simulink model "CODE_GEN"  (R2023b)
settings: Solver=FixedStepDiscrete  StartTime=0.0  StopTime=10.0  FixedStep=0.001  RelTol=1e-3
values from neighbouring files (symbols this model uses):
  alpha = 15/180*pi    (= 0.261799387799)    [MPC_HAC_simulation.m]    (also in init_HAC_simulation.m)
  beta = 50/180*pi    (= 0.872664625997)    [MPC_HAC_simulation.m]    (also in init_HAC_simulation.m)
  E_up = m*g*L*cos(0)    [init_HAC_simulation.m]    (also in init_model.m)
  eta = 1.3    [init_HAC_simulation.m]    (also in init_model.m)
  g = [g; st_next - st_next_RK4]    [MPC_cartPend_casadi.m]    (also in MPC_cartPend_casadi_scaled.m; MPC_casadi_block.m; continuous_cartpend.m = 9.80665; init_HAC_simulation.m = 9.80665)
  I = 8.7395e-04    (= 0.00087395)    [MPC_casadi_block.m]    (also in continuous_cartpend.m = 0.0008739525; init_HAC_simulation.m = 0.0008739525; init_MPC.m = 0.0008739525; init_NMPC.m = 0.0008739525)
  k_cw = 6    [init_HAC_simulation.m]    (also in init_model.m)
  k_em = 10    [init_HAC_simulation.m]    (also in init_model.m)
  k_su = 2    [init_HAC_simulation.m]    (also in init_model.m)
  k_vw = 2.5    [init_HAC_simulation.m]    (also in init_model.m)
  L = 0.1500    (= 0.15)    [MPC_casadi_block.m]    (also in continuous_cartpend.m; init_HAC_simulation.m; init_MPC.m; init_NMPC.m)
  m = 0.116527    [MPC_casadi_block.m]    (also in continuous_cartpend.m; init_HAC_simulation.m; init_MPC.m; init_NMPC.m)
  q_max = 15/180*pi    (= 0.261799387799)    [MPC_HAC_simulation.m]    (also in MPC_cartPend_casadi.m = inf; MPC_cartPend_casadi_scaled.m = 6.28318530718; MPC_casadi_block.m = inf; init_HAC_simulation.m)
  q_min = -q_max    (= -0.261799387799)    [MPC_HAC_simulation.m]    (also in MPC_cartPend_casadi.m = -inf; MPC_cartPend_casadi_scaled.m = -6.28318530718; MPC_casadi_block.m = -inf; init_HAC_simulation.m)
  q_sqm = zeros(1, n_rules_q)    [MPC_HAC_simulation.m]    (also in init_HAC_simulation.m)
  qd_max = inf    [MPC_HAC_simulation.m]    (also in MPC_cartPend_casadi.m; MPC_cartPend_casadi_scaled.m = 13; MPC_casadi_block.m; init_HAC_simulation.m = 5)
  qd_min = -qd_max    (= -inf)    [MPC_HAC_simulation.m]    (also in MPC_cartPend_casadi.m; MPC_cartPend_casadi_scaled.m = -13; MPC_casadi_block.m; init_HAC_simulation.m = -5)
  qd_sqm = zeros(1, n_rules_qd)    [MPC_HAC_simulation.m]    (also in init_HAC_simulation.m)
  u_max = 3 * 9.80665    (= 29.41995)    [MPC_HAC_simulation.m]    (also in MPC_cartPend_casadi.m = 29.43; MPC_cartPend_casadi_scaled.m = 29.43; MPC_casadi_block.m = 29.43; init_HAC_simulation.m)
  u_min = -u_max    (= -29.41995)    [MPC_HAC_simulation.m]    (also in MPC_cartPend_casadi.m = -29.43; MPC_cartPend_casadi_scaled.m = -29.43; MPC_casadi_block.m = -29.43; init_HAC_simulation.m)
  u_q_sqm = zeros(1, n_rules_q)    [MPC_HAC_simulation.m]    (also in init_HAC_simulation.m)
  u_qd_sqm = zeros(1, n_rules_qd)    [MPC_HAC_simulation.m]    (also in init_HAC_simulation.m)
  u_x_sqm = zeros(1, n_rules_x)    [MPC_HAC_simulation.m]    (also in init_HAC_simulation.m)
  u_xd_sqm = zeros(1, n_rules_xd)    [MPC_HAC_simulation.m]    (also in init_HAC_simulation.m)
  uMax = 3*g    (= 29.41995)    [init_HAC_simulation.m]    (also in init_MPC.m; init_NMPC.m; init_model.m)
  w_high = 1    [MPC_HAC_simulation.m]    (also in init_HAC_simulation.m)
  w_low = 0.25    [MPC_HAC_simulation.m]    (also in init_HAC_simulation.m)
  x1_max = 0.43    [init_HAC_simulation.m]    (also in init_MPC.m; init_NMPC.m; init_model.m)
  x2_max = 2    [init_HAC_simulation.m]    (also in init_MPC.m; init_NMPC.m; init_model.m)
  x_max = 0.43    [MPC_HAC_simulation.m]    (also in MPC_cartPend_casadi.m; MPC_cartPend_casadi_scaled.m; MPC_casadi_block.m; init_HAC_simulation.m)
  x_min = -x_max    (= -0.43)    [MPC_HAC_simulation.m]    (also in MPC_cartPend_casadi.m; MPC_cartPend_casadi_scaled.m; MPC_casadi_block.m; init_HAC_simulation.m)
  x_sqm = zeros(1, n_rules_x)    [MPC_HAC_simulation.m]    (also in init_HAC_simulation.m; my_HAC.m = [0 0.00390625 0.0078125 0.01171875 0.015625 0.0234375 0.0312)
  xd_max = 2.0    (= 2)    [MPC_HAC_simulation.m]    (also in MPC_cartPend_casadi.m; MPC_cartPend_casadi_scaled.m; MPC_casadi_block.m; init_HAC_simulation.m)
  xd_min = -xd_max    (= -2)    [MPC_HAC_simulation.m]    (also in MPC_cartPend_casadi.m; MPC_cartPend_casadi_scaled.m; MPC_casadi_block.m; init_HAC_simulation.m)
  xd_sqm = zeros(1, n_rules_xd)    [MPC_HAC_simulation.m]    (also in init_HAC_simulation.m)
libraries: fuzblock x2
settings Model: Creator=doann  LastModifiedBy=doann
settings OptimizationCC: DefaultParameterBehavior=Inlined  UseDivisionForNetSlopeComputation=on  GainParamInheritBuiltInType=on  UseFloatMulNetSlope=on  InlineInvariantSignals=on  PassReuseOutputArgsAs=Individual arguments  ZeroExternalMemoryAtStartup=off  ZeroInternalMemoryAtStartup=off  NoFixptDivByZeroProtection=on  EfficientFloat2IntCast=on  LifeSpan=1  OptimizeBlockOrder=speed  DifferentSizesBufferReuse=on  EfficientTunableParamExpr=on
settings DebuggingCC: ParameterTunabilityLossMsg=error
settings HardwareCC: ProdBitPerPointer=32  ProdBitPerSizeT=32  ProdBitPerPtrDiffT=32  ProdLargestAtomicInteger=Long  ProdLargestAtomicFloat=Double  ProdWordSize=32  ProdLongLongMode=on  ProdHWDeviceType=ARM Compatible->ARM Cortex-M
settings SFSimCC: MATLABDynamicMemAlloc=off
settings RTWCC: Description=Embedded Coder  SystemTargetFile=ert.tlc  TemplateMakefile=ert_default_tmf  TargetLang=C++
settings CodeAppCC: ForceParamTrailComments=on  IgnoreCustomStorageClasses=off  OperatorAnnotations=on  SimulinkDataObjDesc=on  SFDataObjDesc=on  CustomSymbolStrGlobalVar=rt$N$M  CustomSymbolStrType=$N$M  CustomSymbolStrFcn=$N$M$F  CustomSymbolStrMacro=$N$M  InsertBlockDesc=on
settings ERTTargetCC: TargetLangStandard=C++11 (ISO)  GenerateSampleERTMain=on  IncludeMdlTerminateFcn=off  CombineSignalStateStructs=on  SupportAbsoluteTime=off  CodeInterfacePackaging=C++ class  SupportComplex=off  SupportNonInlinedSFcns=on  InlinedParameterPlacement=NonHierarchical  RootIOFormat=Structure reference  ERTCustomFileTemplate=example_file_process.tlc  ERTFilePackagingFormat=CompactWithDataFile

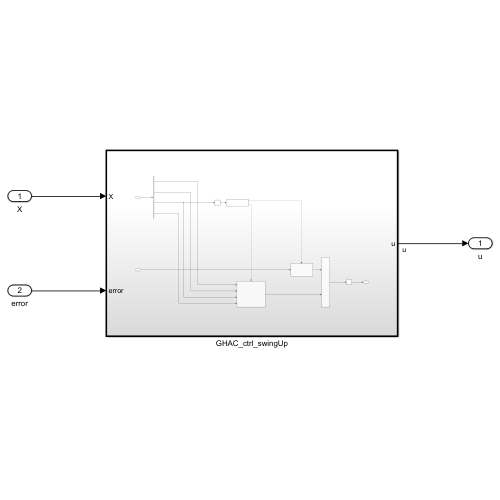
[thumbnail: Simulink's stored preview of the top-level diagram]
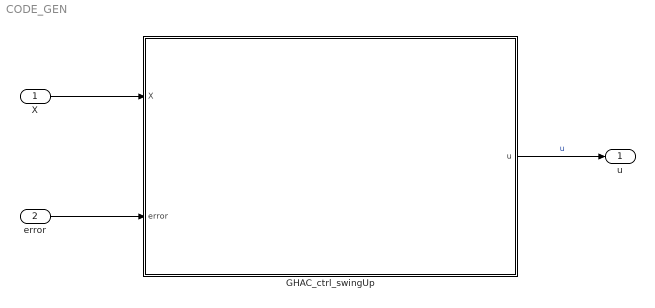
== system CODE_GEN ==
  X : Inport
  error : Inport  Port=2
  GHAC_ctrl_swingUp : Subsystem  TreatAsAtomicUnit=on  SystemSampleTime=0.001
  u : Outport
  wires:
  GHAC_ctrl_swingUp/1(u) -> u/1  "u"
  X/1 -> GHAC_ctrl_swingUp/1(X)
  error/1 -> GHAC_ctrl_swingUp/2(error)

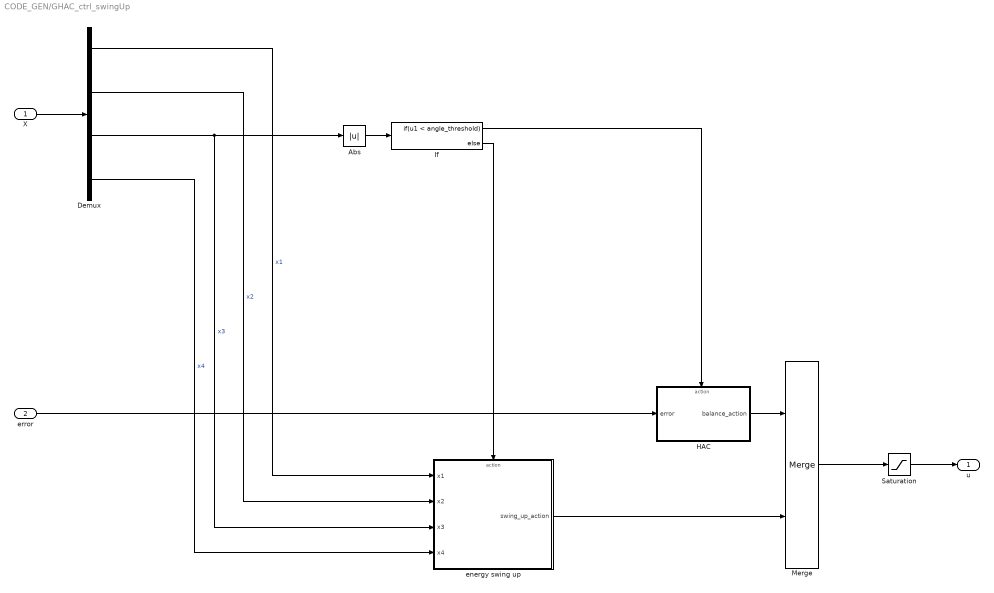
== system CODE_GEN/GHAC_ctrl_swingUp ==
  X : Inport
  error : Inport  Port=2
  Abs : Abs  SaturateOnIntegerOverflow=off
  Demux : Demux
  HAC : Subsystem  TreatAsAtomicUnit=on
  If : If  IfExpression=u1 < angle_threshold
  Merge : Merge
  Saturation : Saturate  UpperLimit=uMax  LowerLimit=-uMax
  energy swing up : Subsystem  TreatAsAtomicUnit=on
  u : Outport
  wires:
  X/1 -> Demux/1
  Demux/3 -> Abs/1, energy swing up/3(x3)  "x3"
  Demux/4 -> energy swing up/4(x4)  "x4"
  Abs/1 -> If/1
  If/1 -> HAC/Action
  If/2 -> energy swing up/Action
  HAC/1(balance_action) -> Merge/1
  energy swing up/1(swing_up_action) -> Merge/2
  error/1 -> HAC/1(error)
  Demux/2 -> energy swing up/2(x2)  "x2"
  Demux/1 -> energy swing up/1(x1)  "x1"
  Merge/1 -> Saturation/1
  Saturation/1 -> u/1

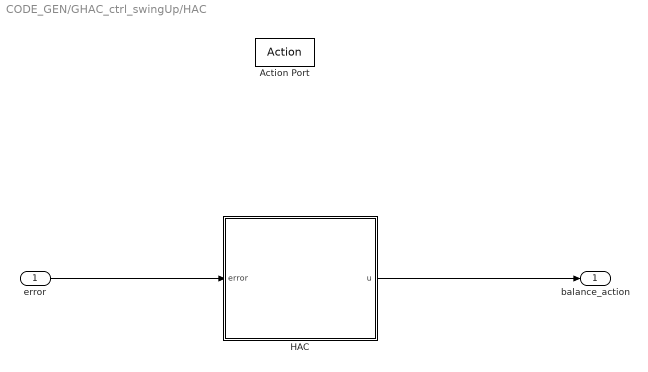
== system CODE_GEN/GHAC_ctrl_swingUp/HAC ==
  error : Inport
  Action Port : ActionPort  ActionPortLabel=if(u1 < angle_threshold)
  HAC : Subsystem
  balance_action : Outport
  wires:
  error/1 -> HAC/1(error)
  HAC/1(u) -> balance_action/1

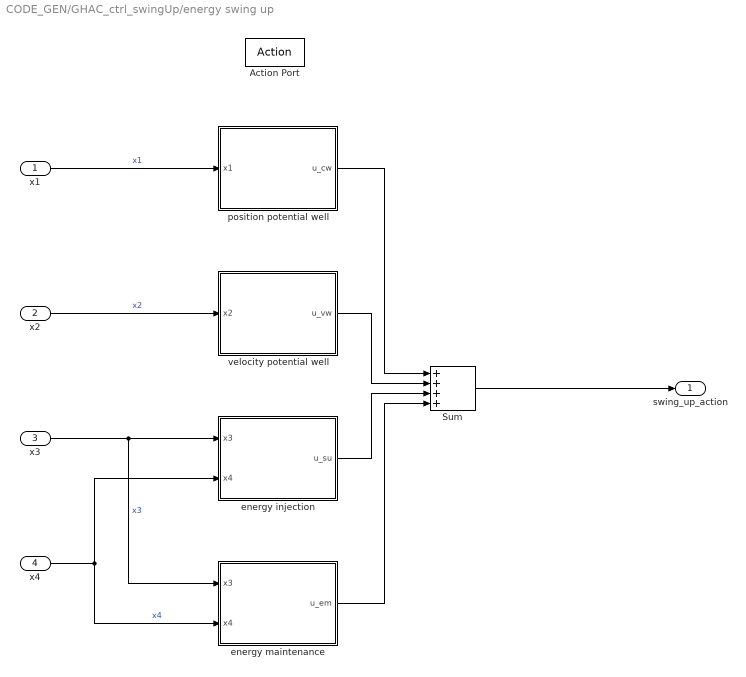
== system CODE_GEN/GHAC_ctrl_swingUp/energy swing up ==
  x1 : Inport
  x2 : Inport  Port=2
  x3 : Inport  Port=3
  x4 : Inport  Port=4
  Action Port : ActionPort  ActionPortLabel=else
  Sum : Sum  Inputs=++++
  energy injection : Subsystem
  energy maintenance : Subsystem
  position potential well : Subsystem
  velocity potential well : Subsystem
  swing_up_action : Outport
  wires:
  energy injection/1(u_su) -> Sum/3
  x2/1 -> velocity potential well/1(x2)  "x2"
  velocity potential well/1(u_vw) -> Sum/2
  Sum/1 -> swing_up_action/1
  energy maintenance/1(u_em) -> Sum/4
  x3/1 -> energy maintenance/1(x3), energy injection/1(x3)  "x3"
  x1/1 -> position potential well/1(x1)  "x1"
  x4/1 -> energy injection/2(x4), energy maintenance/2(x4)  "x4"
  position potential well/1(u_cw) -> Sum/1

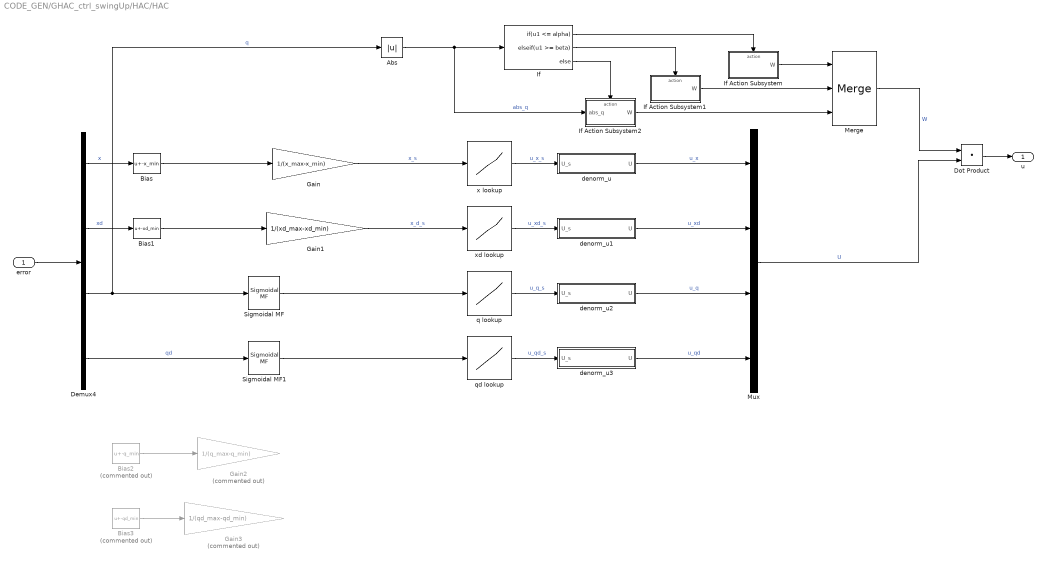
== system CODE_GEN/GHAC_ctrl_swingUp/HAC/HAC ==
  error : Inport
  Abs : Abs  SaturateOnIntegerOverflow=off
  Bias : Bias  Bias=-x_min  SaturateOnIntegerOverflow=off
  Bias1 : Bias  Bias=-xd_min  SaturateOnIntegerOverflow=off
  Bias2 : Bias  Commented=on  Bias=-q_min  SaturateOnIntegerOverflow=off
  Bias3 : Bias  Commented=on  Bias=-qd_min  SaturateOnIntegerOverflow=off
  Demux4 : Demux
  Dot Product : DotProduct  OutDataTypeStr=Inherit: Inherit via internal rule
  Gain : Gain  Gain=1/(x_max-x_min)
  Gain1 : Gain  Gain=1/(xd_max-xd_min)
  Gain2 : Gain  Commented=on  Gain=1/(q_max-q_min)
  Gain3 : Gain  Commented=on  Gain=1/(qd_max-qd_min)
  If : If  IfExpression=u1 <= alpha  ElseIfExpressions=u1 >= beta
  If Action Subsystem : Subsystem  TreatAsAtomicUnit=on
  If Action Subsystem1 : Subsystem  TreatAsAtomicUnit=on
  If Action Subsystem2 : Subsystem  TreatAsAtomicUnit=on
  Merge : Merge  Inputs=3
  Mux : Mux
  Sigmoidal MF : fuzblock/Membership  Functions/Sigmoidal MF  a=a_sigmoid_q  c=0
  Sigmoidal MF1 : fuzblock/Membership  Functions/Sigmoidal MF  a=a_sigmoid_q_d  c=0
  denorm_u : Subsystem
  denorm_u1 : Subsystem
  denorm_u2 : Subsystem
  denorm_u3 : Subsystem
  q lookup : Lookup_n-D  NumberOfTableDimensions=1  BreakpointsForDimension1=q_sqm  Table=u_q_sqm  InternalRulePriority=Speed  RndMeth=Simplest
  qd lookup : Lookup_n-D  NumberOfTableDimensions=1  BreakpointsForDimension1=qd_sqm  Table=u_qd_sqm  InternalRulePriority=Speed  RndMeth=Simplest
  x lookup : Lookup_n-D  NumberOfTableDimensions=1  BreakpointsForDimension1=x_sqm  Table=u_x_sqm  InternalRulePriority=Speed  RndMeth=Simplest
  xd lookup : Lookup_n-D  NumberOfTableDimensions=1  BreakpointsForDimension1=xd_sqm  Table=u_xd_sqm  InternalRulePriority=Speed  RndMeth=Simplest
  u : Outport
  wires:
  Demux4/3 -> Sigmoidal MF/1, Abs/1  "q"
  Gain/1 -> x lookup/1  "x_s"
  Abs/1 -> If Action Subsystem2/1(abs_q), If/1  "abs_q"
  If/1 -> If Action Subsystem/Action
  If/2 -> If Action Subsystem1/Action
  If/3 -> If Action Subsystem2/Action
  If Action Subsystem/1(W) -> Merge/1
  If Action Subsystem1/1(W) -> Merge/2
  If Action Subsystem2/1(W) -> Merge/3
  Dot Product/1 -> u/1
  error/1 -> Demux4/1
  Bias/1 -> Gain/1
  Demux4/1 -> Bias/1  "x"
  Bias1/1 -> Gain1/1
  Gain1/1 -> xd lookup/1  "x_d_s"
  Demux4/2 -> Bias1/1  "xd"
  Bias2/1 -> Gain2/1
  Bias3/1 -> Gain3/1
  x lookup/1 -> denorm_u/1(U_s)  "u_x_s"
  denorm_u/1(U) -> Mux/1  "u_x"
  xd lookup/1 -> denorm_u1/1(U_s)  "u_xd_s"
  denorm_u1/1(U) -> Mux/2  "u_xd"
  q lookup/1 -> denorm_u2/1(U_s)  "u_q_s"
  denorm_u2/1(U) -> Mux/3  "u_q"
  qd lookup/1 -> denorm_u3/1(U_s)  "u_qd_s"
  denorm_u3/1(U) -> Mux/4  "u_qd"
  Mux/1 -> Dot Product/2  "U"
  Sigmoidal MF/1 -> q lookup/1
  Sigmoidal MF1/1 -> qd lookup/1
  Demux4/4 -> Sigmoidal MF1/1  "qd"
  Merge/1 -> Dot Product/1  "W"

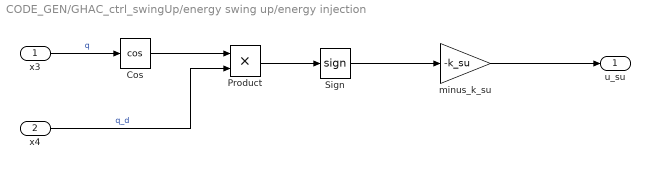
== system CODE_GEN/GHAC_ctrl_swingUp/energy swing up/energy injection ==
  x3 : Inport
  x4 : Inport  Port=2
  Cos : Trigonometry  Operator=cos
  Product : Product
  Sign : Signum
  minus_k_su : Gain  Gain=-k_su
  u_su : Outport
  wires:
  x3/1 -> Cos/1  "q"
  x4/1 -> Product/2  "q_d"
  Sign/1 -> minus_k_su/1
  minus_k_su/1 -> u_su/1
  Cos/1 -> Product/1
  Product/1 -> Sign/1

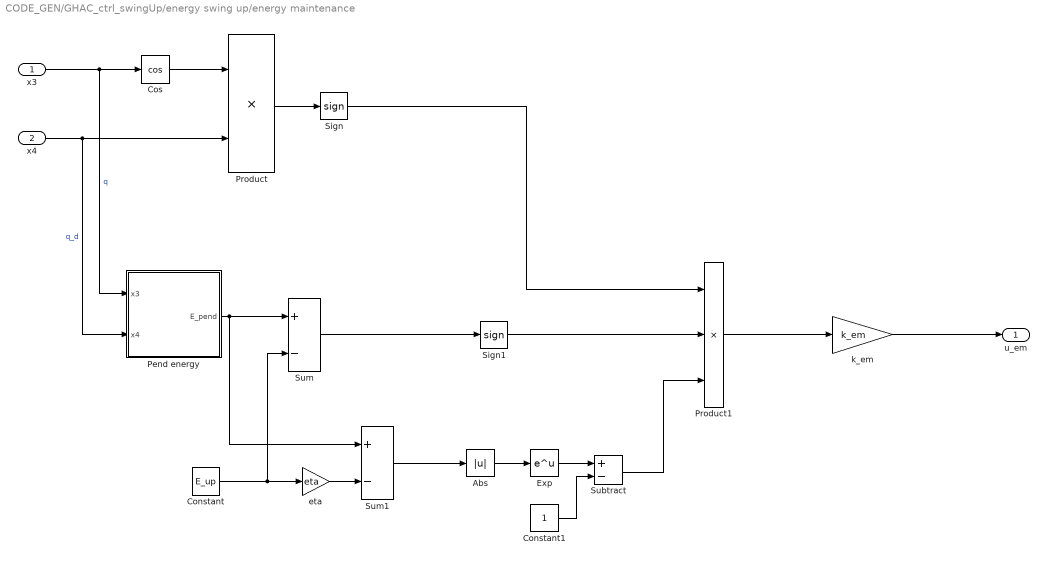
== system CODE_GEN/GHAC_ctrl_swingUp/energy swing up/energy maintenance ==
  x3 : Inport
  x4 : Inport  Port=2
  Abs : Abs  SaturateOnIntegerOverflow=off
  Constant : Constant  Value=E_up
  Constant1 : Constant
  Cos : Trigonometry  Operator=cos
  Exp : Math
  Pend energy : Subsystem
  Product : Product
  Product1 : Product  Inputs=3
  Sign : Signum
  Sign1 : Signum
  Subtract : Sum  Inputs=+-
  Sum : Sum  Inputs=+-
  Sum1 : Sum  Inputs=+-
  eta : Gain  Gain=eta
  k_em : Gain  Gain=k_em
  u_em : Outport
  wires:
  x3/1 -> Pend energy/1(x3), Cos/1  "q"
  Cos/1 -> Product/1
  x4/1 -> Pend energy/2(x4), Product/2  "q_d"
  Product/1 -> Sign/1
  Pend energy/1(E_pend) -> Sum/1, Sum1/1
  Constant/1 -> Sum/2, eta/1
  Sum/1 -> Sign1/1
  eta/1 -> Sum1/2
  Sum1/1 -> Abs/1
  Abs/1 -> Exp/1
  Exp/1 -> Subtract/1
  Constant1/1 -> Subtract/2
  Sign1/1 -> Product1/2
  Sign/1 -> Product1/1
  Subtract/1 -> Product1/3
  Product1/1 -> k_em/1
  k_em/1 -> u_em/1

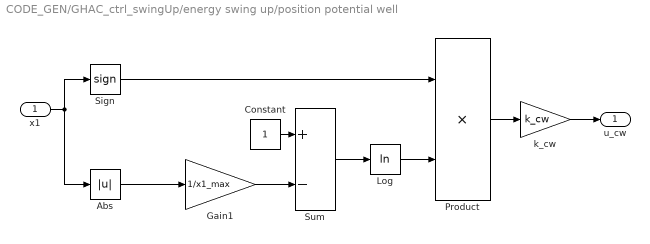
== system CODE_GEN/GHAC_ctrl_swingUp/energy swing up/position potential well ==
  x1 : Inport
  Abs : Abs  SaturateOnIntegerOverflow=off
  Constant : Constant
  Gain1 : Gain  Gain=1/x1_max
  Log : Math  Operator=log
  Product : Product
  Sign : Signum
  Sum : Sum  Inputs=+-
  k_cw : Gain  Gain=k_cw
  u_cw : Outport
  wires:
  x1/1 -> Abs/1, Sign/1
  Abs/1 -> Gain1/1
  Gain1/1 -> Sum/2
  Constant/1 -> Sum/1
  Sum/1 -> Log/1
  k_cw/1 -> u_cw/1
  Product/1 -> k_cw/1
  Log/1 -> Product/2
  Sign/1 -> Product/1

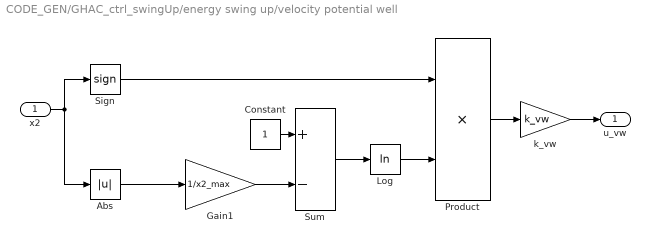
== system CODE_GEN/GHAC_ctrl_swingUp/energy swing up/velocity potential well ==
  x2 : Inport
  Abs : Abs  SaturateOnIntegerOverflow=off
  Constant : Constant
  Gain1 : Gain  Gain=1/x2_max
  Log : Math  Operator=log
  Product : Product
  Sign : Signum
  Sum : Sum  Inputs=+-
  k_vw : Gain  Gain=k_vw
  u_vw : Outport
  wires:
  Sign/1 -> Product/1
  Log/1 -> Product/2
  Product/1 -> k_vw/1
  k_vw/1 -> u_vw/1
  Sum/1 -> Log/1
  Constant/1 -> Sum/1
  Gain1/1 -> Sum/2
  Abs/1 -> Gain1/1
  x2/1 -> Sign/1, Abs/1

== system CODE_GEN/GHAC_ctrl_swingUp/HAC/HAC/If Action Subsystem ==
  Action Port : ActionPort  ActionPortLabel=if(u1 <= alpha)
  weight : Constant  Value=[0.25; 0.25; 0.25; 0.25]  VectorParams1D=off
  W : Outport
  wires:
  weight/1 -> W/1

== system CODE_GEN/GHAC_ctrl_swingUp/HAC/HAC/If Action Subsystem1 ==
  Action Port : ActionPort  ActionPortLabel=elseif(u1 >= beta)
  weights : Constant  Value=[0; 0; 1; 0]  VectorParams1D=off
  W : Outport
  wires:
  weights/1 -> W/1

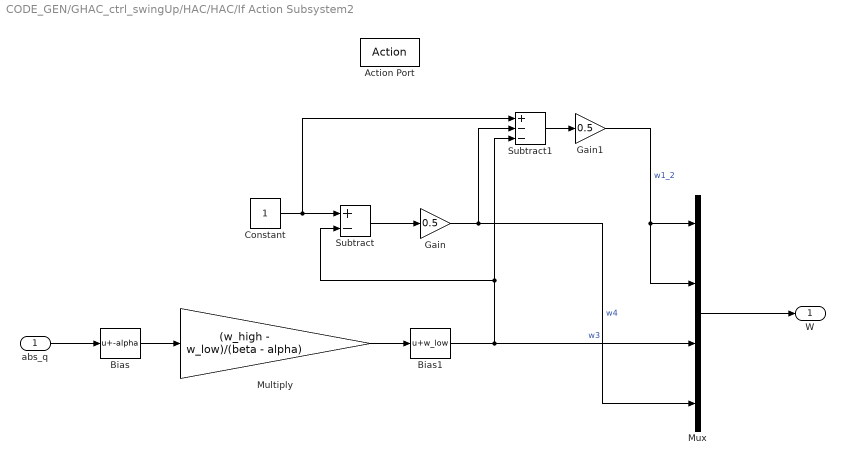
== system CODE_GEN/GHAC_ctrl_swingUp/HAC/HAC/If Action Subsystem2 ==
  abs_q : Inport
  Action Port : ActionPort  ActionPortLabel=else
  Bias : Bias  Bias=-alpha  SaturateOnIntegerOverflow=off
  Bias1 : Bias  Bias=w_low  SaturateOnIntegerOverflow=off
  Constant : Constant
  Gain : Gain  Gain=0.5
  Gain1 : Gain  Gain=0.5
  Multiply : Gain  Gain=(w_high - w_low)/(beta - alpha)
  Mux : Mux
  Subtract : Sum  Inputs=+-
  Subtract1 : Sum  Inputs=+--
  W : Outport
  wires:
  Mux/1 -> W/1
  abs_q/1 -> Bias/1
  Bias/1 -> Multiply/1
  Multiply/1 -> Bias1/1
  Bias1/1 -> Subtract/2, Subtract1/3, Mux/3  "w3"
  Constant/1 -> Subtract1/1, Subtract/1
  Subtract/1 -> Gain/1
  Gain/1 -> Subtract1/2, Mux/4  "w4"
  Subtract1/1 -> Gain1/1
  Gain1/1 -> Mux/1, Mux/2  "w1_2"

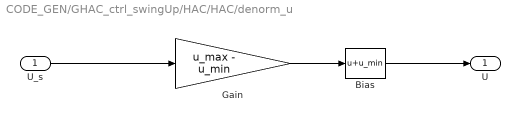
== system CODE_GEN/GHAC_ctrl_swingUp/HAC/HAC/denorm_u ==
  U_s : Inport
  Bias : Bias  Bias=u_min  SaturateOnIntegerOverflow=off
  Gain : Gain  Gain=u_max - u_min
  U : Outport
  wires:
  U_s/1 -> Gain/1
  Gain/1 -> Bias/1
  Bias/1 -> U/1

== system CODE_GEN/GHAC_ctrl_swingUp/HAC/HAC/denorm_u1 ==
  U_s : Inport
  Bias : Bias  Bias=u_min  SaturateOnIntegerOverflow=off
  Gain : Gain  Gain=u_max - u_min
  U : Outport
  wires:
  Bias/1 -> U/1
  Gain/1 -> Bias/1
  U_s/1 -> Gain/1

== system CODE_GEN/GHAC_ctrl_swingUp/HAC/HAC/denorm_u2 ==
  U_s : Inport
  Bias : Bias  Bias=u_min  SaturateOnIntegerOverflow=off
  Gain : Gain  Gain=u_max - u_min
  U : Outport
  wires:
  U_s/1 -> Gain/1
  Gain/1 -> Bias/1
  Bias/1 -> U/1

== system CODE_GEN/GHAC_ctrl_swingUp/HAC/HAC/denorm_u3 ==
  U_s : Inport
  Bias : Bias  Bias=u_min  SaturateOnIntegerOverflow=off
  Gain : Gain  Gain=u_max - u_min
  U : Outport
  wires:
  Bias/1 -> U/1
  Gain/1 -> Bias/1
  U_s/1 -> Gain/1

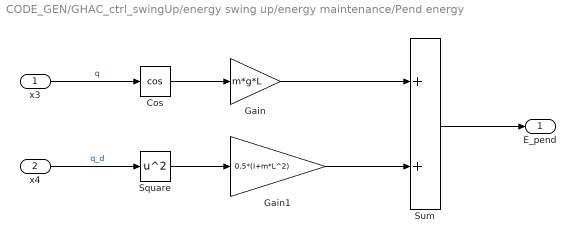
== system CODE_GEN/GHAC_ctrl_swingUp/energy swing up/energy maintenance/Pend energy ==
  x3 : Inport
  x4 : Inport  Port=2
  Cos : Trigonometry  Operator=cos
  Gain : Gain  Gain=m*g*L
  Gain1 : Gain  Gain=0.5*(I+m*L^2)
  Square : Math  Operator=square
  Sum : Sum
  E_pend : Outport
  wires:
  x3/1 -> Cos/1  "q"
  x4/1 -> Square/1  "q_d"
  Cos/1 -> Gain/1
  Square/1 -> Gain1/1
  Gain/1 -> Sum/1
  Gain1/1 -> Sum/2
  Sum/1 -> E_pend/1
